simulink model "chap8_6sim"  (Simulink 7.7)
settings: Solver=ode45  StartTime=0.0  StopTime=1  FixedStep=0.001  RelTol=1e-3
settings Model: Creator=hp  LastModifiedBy=ljk
settings DataIOCC: SignalLoggingName=sigsOut
settings OptimizationCC: InitFltsAndDblsToZero=on
settings DebuggingCC: SaveWithParameterizedLinksMsg=none  SignalResolutionControl=TryResolveAllWithWarning  SolverPrmCheckMsg=none  MultiTaskDSMMsg=warning  MultiTaskCondExecSysMsg=none  StrictBusMsg=Warning
settings HardwareCC: TargetUnknown=on
settings RTWCC: IncludeERTFirstTime=on
settings GRTTargetCC: TargetFcnLib=ansi_tfl_tmw.mat

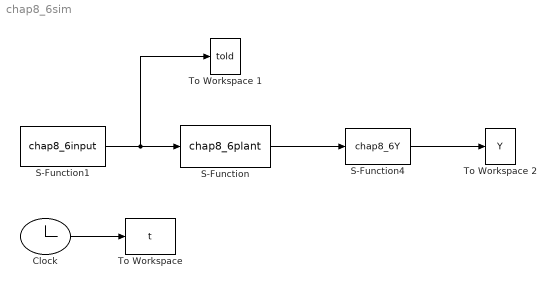
== system chap8_6sim ==
  Clock : Clock
      settings: Decimation=10
  S-Function : S-Function  FunctionName=chap8_6plant  EnableBusSupport=off
  S-Function1 : S-Function  FunctionName=chap8_6input  EnableBusSupport=off
  S-Function4 : S-Function  FunctionName=chap8_6Y  EnableBusSupport=off
  To Workspace : ToWorkspace  VariableName=t  SampleTime=-1  SaveFormat=Array
  To Workspace 1 : ToWorkspace  VariableName=told  SampleTime=-1  SaveFormat=Array
  To Workspace 2 : ToWorkspace  VariableName=Y  SampleTime=-1  SaveFormat=Array
  wires:
  Clock/1 -> To Workspace/1
  S-Function1/1 -> S-Function/1, To Workspace 1/1
  S-Function/1 -> S-Function4/1
  S-Function4/1 -> To Workspace 2/1
